simulink library "ccslrel"  (R2017a)
settings: Solver=VariableStepAuto  StartTime=0.0  StopTime=10.0  RelTol=1e-3
libraries: sldvlib x5
settings Model: Creator=Li  LastModifiedBy=Li

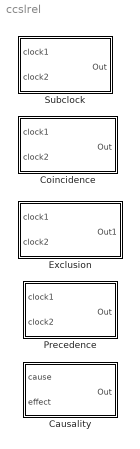
== system ccslrel ==
  " Causality" : Subsystem  mask(Causality){}
      mask help: This block checks whether one clock runs not slower than the other clock, i.e., the cause clock must happen prior to or simultaneously with the effect clock. If this relation is satified, the output of the block will be true; otherwise it will be false.
  Coincidence : Subsystem  mask(Coincidence){}
      mask help: This block checks the coincidence relation between two clocks: clock1 and clock2. Two clocks are coincident if the steps at which the value of one clock is true, the other is also true. If clock1 is coincident with clock2, the output will be true. Otherwise it will be false.
  Exclusion : Subsystem  mask(Exclusion){}
      mask help: This block checks whether two clocks exclude each other, i.e., two clocks do not tick at the same step. If the exclusion relation holds, the output of the clock will be true. Otherwise it will be false.
  Precedence : Subsystem  mask(Precedence){}
      mask help: This block checks whether one clock precedes the other, i.e., clock1 precedes clock2. If the precedence relation holds between clock1 and clock2, the output of this block will be true. Otherwise it will be false.
  Subclock : Subsystem  mask(Subclock){}
      mask help: This block checks whether one clock is the subclock of the other, i.e., clock1 is the subclock of clock2. It will return true if the subclock relation is satisfied. Otherwise it will return false.

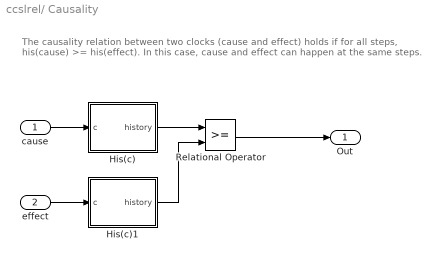
== system ccslrel/ Causality ==
  note: The causality relation between two clocks (cause and effect) holds if for all steps, his(cause) >= his(effect). In this case, cause and effect can happen at the same steps.
  cause : Inport
  effect : Inport  Port=2
  His(c) : Subsystem
  His(c)1 : Subsystem
  Relational Operator : RelationalOperator  OutDataTypeStr=boolean  RndMeth=Simplest
  Out : Outport
  wires:
  effect/1 -> His(c)1/1(c)
  His(c)/1(history) -> Relational Operator/1
  His(c)1/1(history) -> Relational Operator/2
  cause/1 -> His(c)/1(c)
  Relational Operator/1 -> Out/1

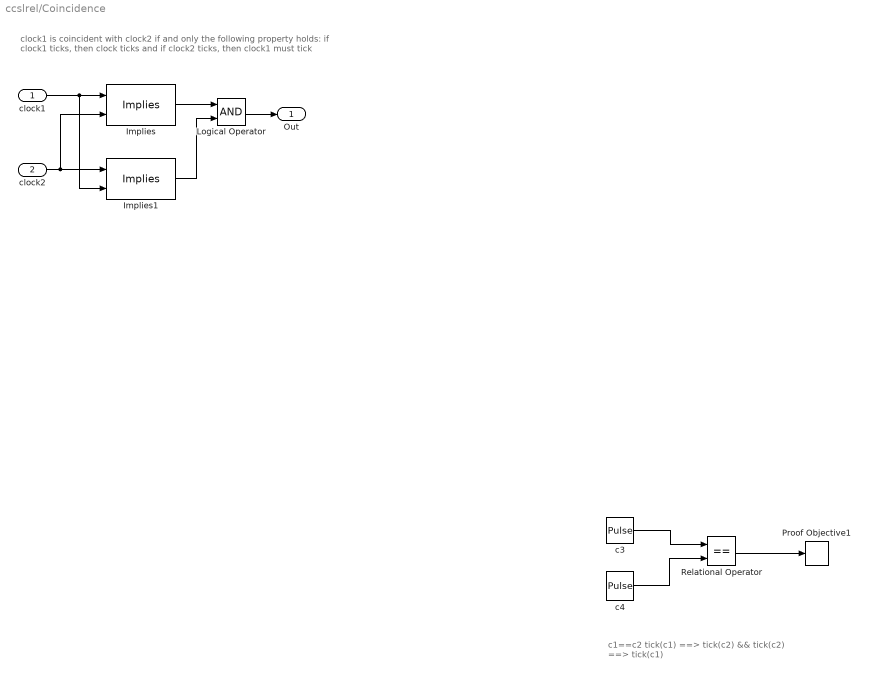
== system ccslrel/Coincidence ==
  note: clock1 is coincident with clock2 if and only the following property holds:
      | if clock1 ticks, then clock ticks and if clock2 ticks, then clock1 must tick
  note: c1==c2
      | tick(c1) ==> tick(c2) && tick(c2) ==> tick(c1)
  clock1 : Inport
  clock2 : Inport  Port=2
  Implies : sldvlib/Verification Utilities/Implies
      settings: SourceProductName=Simulink Design Verifier  SourceProductBaseCode=DV
  Implies1 : sldvlib/Verification Utilities/Implies
      settings: SourceProductName=Simulink Design Verifier  SourceProductBaseCode=DV
  Logical Operator : Logic  AllPortsSameDT=off  OutDataTypeStr=boolean
  Proof Objective1 : sldvlib/Objectives and Constraints/Proof Objective  enabled=on  customAVTBlockType=Proof Objective  intervals=true  dispValues=on  outEnabled=on  enableStopSim=off
      settings: AttributesFormatString=%<intervals>  SourceProductName=Simulink Design Verifier  SourceProductBaseCode=DV
  Relational Operator : RelationalOperator  Operator===  OutDataTypeStr=boolean  RndMeth=Simplest
  c3 : DiscretePulseGenerator  PulseType=Time based  Period=10  PulseWidth=10  PhaseDelay=1
  c4 : DiscretePulseGenerator  PulseType=Time based  Period=10  PulseWidth=10  PhaseDelay=1
  Out : Outport
  wires:
  clock1/1 -> Implies1/2, Implies/1
  Relational Operator/1 -> Proof Objective1/1
  Implies1/1 -> Logical Operator/2
  c3/1 -> Relational Operator/1
  Implies/1 -> Logical Operator/1
  c4/1 -> Relational Operator/2
  clock2/1 -> Implies/2, Implies1/1
  Logical Operator/1 -> Out/1

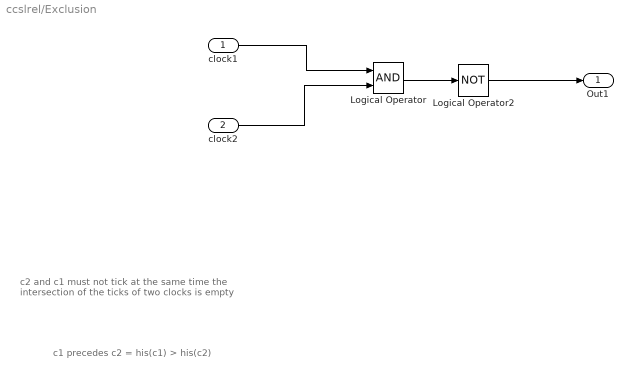
== system ccslrel/Exclusion ==
  note: c2 and c1 must not tick at the same time
      | the intersection of the ticks of two clocks is empty
  note: c1 precedes c2 = his(c1) > his(c2)
  clock1 : Inport
  clock2 : Inport  Port=2
  Logical Operator : Logic  AllPortsSameDT=off  OutDataTypeStr=boolean
  Logical Operator2 : Logic  Operator=NOT  AllPortsSameDT=off  OutDataTypeStr=boolean
  Out1 : Outport
  wires:
  Logical Operator/1 -> Logical Operator2/1
  clock1/1 -> Logical Operator/1
  clock2/1 -> Logical Operator/2
  Logical Operator2/1 -> Out1/1

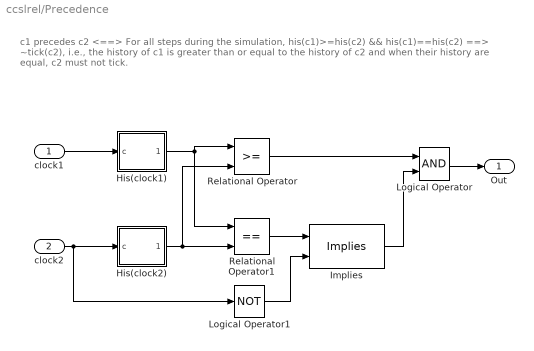
== system ccslrel/Precedence ==
  note: c1 precedes c2 <==> For all steps during the simulation, his(c1)>=his(c2) && his(c1)==his(c2) ==> ~tick(c2), i.e., the history of c1 is greater than or equal to the history of c2 and when their history
      | are equal, c2 must not tick.
  clock1 : Inport
  clock2 : Inport  Port=2
  His(clock1) : Subsystem
  His(clock2) : Subsystem
  Implies : sldvlib/Verification Utilities/Implies
      settings: SourceProductName=Simulink Design Verifier  SourceProductBaseCode=DV
  Logical Operator : Logic  AllPortsSameDT=off  OutDataTypeStr=boolean
  Logical Operator1 : Logic  Operator=NOT  AllPortsSameDT=off  OutDataTypeStr=boolean
  Relational Operator : RelationalOperator  OutDataTypeStr=boolean  RndMeth=Simplest
  Relational Operator1 : RelationalOperator  Operator===  OutDataTypeStr=boolean  RndMeth=Simplest
  Out : Outport
  wires:
  Relational Operator1/1 -> Implies/1
  His(clock2)/1(history) -> Relational Operator/2, Relational Operator1/2
  His(clock1)/1(history) -> Relational Operator/1, Relational Operator1/1
  clock1/1 -> His(clock1)/1(c)
  clock2/1 -> Logical Operator1/1, His(clock2)/1(c)
  Logical Operator1/1 -> Implies/2
  Relational Operator/1 -> Logical Operator/1
  Implies/1 -> Logical Operator/2
  Logical Operator/1 -> Out/1

== system ccslrel/Subclock ==
  note: clock1 is a subclock of clock2 if and only if for all steps, tick(clock1) ==> tick(clock2), i.e., whenever clock1 ticks, clock2 must tick at the same time step. In other words, clock2 is the superclock of clock1.
  clock1 : Inport
  clock2 : Inport  Port=2
  Implies : sldvlib/Verification Utilities/Implies
      settings: SourceProductName=Simulink Design Verifier  SourceProductBaseCode=DV
  Out : Outport
  wires:
  clock1/1 -> Implies/1
  clock2/1 -> Implies/2
  Implies/1 -> Out/1

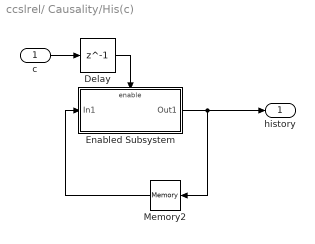
== system ccslrel/ Causality/His(c) ==
  c : Inport
  Delay : Delay  DelayLength=1  InitialCondition=0
  Enabled Subsystem : Subsystem  TreatAsAtomicUnit=on
  Memory2 : Memory
  history : Outport
  wires:
  c/1 -> Delay/1
  Delay/1 -> Enabled Subsystem/Enable
  Enabled Subsystem/1(Out1) -> history/1, Memory2/1
  Memory2/1 -> Enabled Subsystem/1(In1)

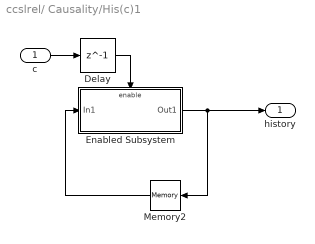
== system ccslrel/ Causality/His(c)1 ==
  c : Inport
  Delay : Delay  DelayLength=1  InitialCondition=0
  Enabled Subsystem : Subsystem  TreatAsAtomicUnit=on
  Memory2 : Memory
  history : Outport
  wires:
  Memory2/1 -> Enabled Subsystem/1(In1)
  Enabled Subsystem/1(Out1) -> Memory2/1, history/1
  Delay/1 -> Enabled Subsystem/Enable
  c/1 -> Delay/1

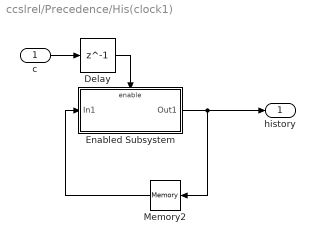
== system ccslrel/Precedence/His(clock1) ==
  c : Inport
  Delay : Delay  DelayLength=1  InitialCondition=0
  Enabled Subsystem : Subsystem  TreatAsAtomicUnit=on
  Memory2 : Memory
  history : Outport
  wires:
  c/1 -> Delay/1
  Delay/1 -> Enabled Subsystem/Enable
  Enabled Subsystem/1(Out1) -> history/1, Memory2/1
  Memory2/1 -> Enabled Subsystem/1(In1)

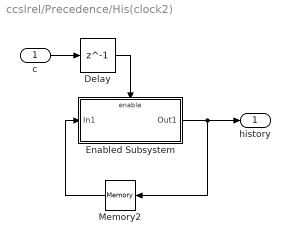
== system ccslrel/Precedence/His(clock2) ==
  c : Inport
  Delay : Delay  DelayLength=1  InitialCondition=0
  Enabled Subsystem : Subsystem  TreatAsAtomicUnit=on
  Memory2 : Memory
  history : Outport
  wires:
  Memory2/1 -> Enabled Subsystem/1(In1)
  Enabled Subsystem/1(Out1) -> history/1, Memory2/1
  Delay/1 -> Enabled Subsystem/Enable
  c/1 -> Delay/1

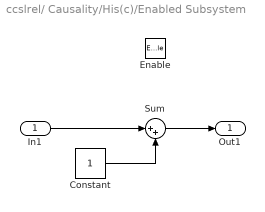
== system ccslrel/ Causality/His(c)/Enabled Subsystem ==
  In1 : Inport
  Enable : EnablePort
  Constant : Constant
  Sum : Sum  Inputs=|++
  Out1 : Outport
  wires:
  In1/1 -> Sum/1
  Constant/1 -> Sum/2
  Sum/1 -> Out1/1

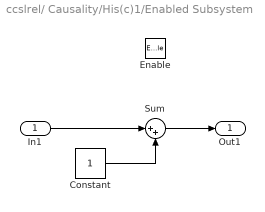
== system ccslrel/ Causality/His(c)1/Enabled Subsystem ==
  In1 : Inport
  Enable : EnablePort
  Constant : Constant
  Sum : Sum  Inputs=|++
  Out1 : Outport
  wires:
  Sum/1 -> Out1/1
  Constant/1 -> Sum/2
  In1/1 -> Sum/1

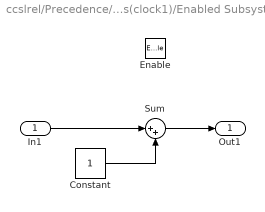
== system ccslrel/Precedence/His(clock1)/Enabled Subsystem ==
  In1 : Inport
  Enable : EnablePort
  Constant : Constant
  Sum : Sum  Inputs=|++
  Out1 : Outport
  wires:
  In1/1 -> Sum/1
  Constant/1 -> Sum/2
  Sum/1 -> Out1/1

== system ccslrel/Precedence/His(clock2)/Enabled Subsystem ==
  In1 : Inport
  Enable : EnablePort
  Constant : Constant
  Sum : Sum  Inputs=|++
  Out1 : Outport
  wires:
  Sum/1 -> Out1/1
  Constant/1 -> Sum/2
  In1/1 -> Sum/1
